simulink model "temp_control_system"  (R2023b)
settings: Solver=VariableStepAuto  StartTime=0.0  StopTime=10  RelTol=1e-3
values from neighbouring files (symbols this model uses):
  Ku = 1    [TEMPPARA.m]
  tau = 10    [TEMPPARA.m]
settings Model: Creator=ascom  LastModifiedBy=ascom

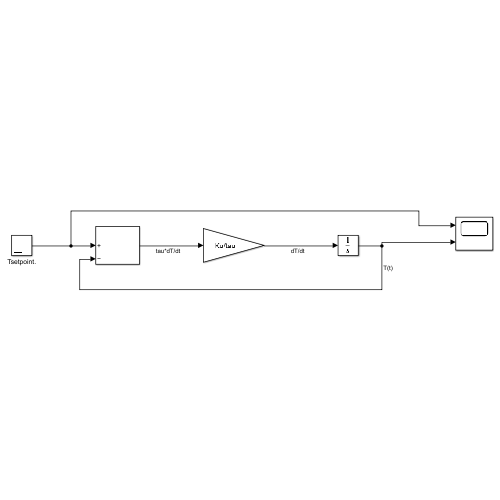
[thumbnail: Simulink's stored preview of the top-level diagram]
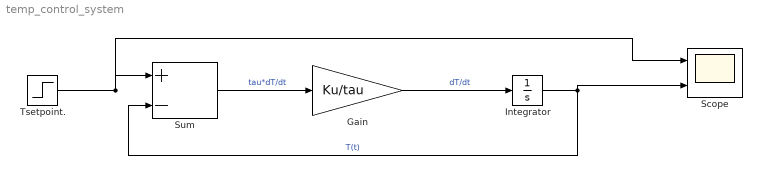
== system temp_control_system ==
  Gain : Gain  Gain=Ku/tau
  Integrator : Integrator
  Scope : Scope  NumInputPorts=2
  Sum : Sum  Inputs=|+-
  Tsetpoint. : Step  SampleTime=0
  wires:
  Sum/1 -> Gain/1  "tau*dT/dt"
  Gain/1 -> Integrator/1  "dT/dt"
  Integrator/1 -> Sum/2, Scope/2  "T(t)"
  Tsetpoint./1 -> Scope/1, Sum/1
